simulink model "A4D_LQR"  (R2016a)
settings: Solver=VariableStepAuto  StartTime=0.0  StopTime=10.0  RelTol=1e-3
values from neighbouring files (symbols this model uses):
  A = [Y_Beta/u Y_p/u -(1-Y_r/u) g*cos(0.0872)/u ... (first row only)    [lateral.m]    (also in longitudinal.m = [X_u  X_w 0 -g; Z_u Z_w u 0; M_u+M_w_dot*Z_u M_w+M_w_dot*Z_w; rscale.m = a)
  B = [0 Y_Delta_r ... (first row only)    [lateral.m]    (also in longitudinal.m = [0; 0; M_delta+M_wdot*Z_delta; 0]; rscale.m = b)
  C = I    [lateral.m]    (also in longitudinal.m = [0 0 0 -1]; rscale.m = c)
undefined symbols (not defined in the file or in its folder): Kgain
settings Model: Creator=kumabhi  LastModifiedBy=kumabhi

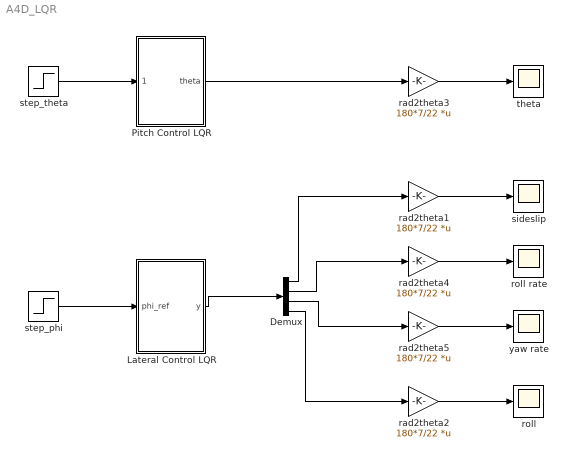
== system A4D_LQR ==
  Demux : Demux
  Lateral Control LQR : Subsystem
      mask Display: image('/home/kumabhi/Pictures/aircraft.png');
  Pitch Control LQR : Subsystem
      mask Display: image('/home/kumabhi/Pictures/aircraft.png');
  rad2theta{1..5} (5 alike) : Gain  Gain=180*7/22  Multiplication=Matrix(K*u)
  roll : Scope
  roll rate : Scope
  sideslip : Scope
  step_phi : Step  After=1.0472  SampleTime=0
  step_theta : Step  After=0.0872665  SampleTime=0
  theta : Scope
  yaw rate : Scope
  wires:
  step_theta/1 -> Pitch Control LQR/1(theta_ref)
  Pitch Control LQR/1(theta) -> rad2theta3/1
  step_phi/1 -> Lateral Control LQR/1(phi_ref)
  Lateral Control LQR/1(y) -> Demux/1
  Demux/1 -> rad2theta1/1
  rad2theta2/1 -> roll/1
  rad2theta1/1 -> sideslip/1
  rad2theta3/1 -> theta/1
  Demux/4 -> rad2theta2/1
  Demux/2 -> rad2theta4/1
  rad2theta4/1 -> roll rate/1
  Demux/3 -> rad2theta5/1
  rad2theta5/1 -> yaw rate/1

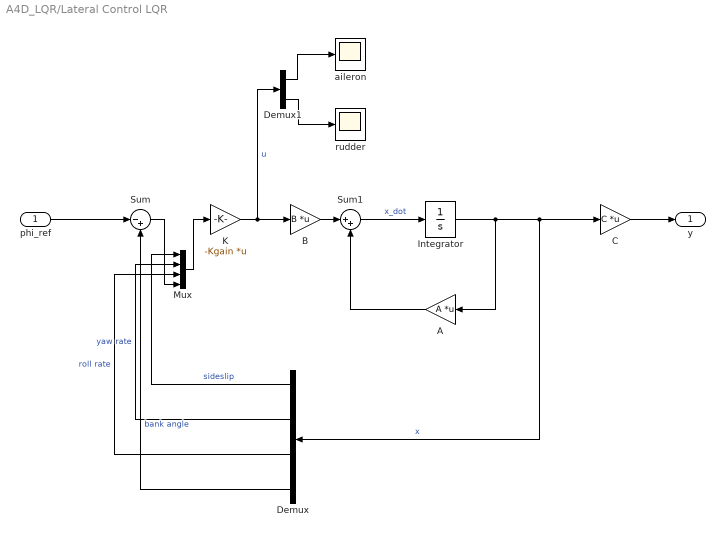
== system A4D_LQR/Lateral Control LQR ==
  phi_ref : Inport
  A : Gain  Gain=A  Multiplication=Matrix(K*u)
  B : Gain  Gain=B  Multiplication=Matrix(K*u)
  C : Gain  Gain=C  Multiplication=Matrix(K*u)
  Demux : Demux
  Demux1 : Demux  Outputs=2
  Integrator : Integrator
  K : Gain  Gain=-Kgain  Multiplication=Matrix(K*u)
  Mux : Mux
  Sum : Sum  Inputs=|-+
  Sum1 : Sum  Inputs=|++
  aileron : Scope
  rudder : Scope
  y : Outport
  wires:
  Integrator/1 -> A/1, Demux/1, C/1  "x"
  A/1 -> Sum1/2
  Sum1/1 -> Integrator/1  "x_dot"
  C/1 -> y/1
  phi_ref/1 -> Sum/1
  B/1 -> Sum1/1
  Demux/2 -> Mux/2  "yaw rate"
  Demux/3 -> Mux/3  "roll rate"
  Demux/4 -> Sum/2  "bank angle"
  Sum/1 -> Mux/4
  Mux/1 -> K/1
  K/1 -> Demux1/1, B/1  "u"
  Demux1/1 -> aileron/1
  Demux1/2 -> rudder/1
  Demux/1 -> Mux/1  "sideslip"

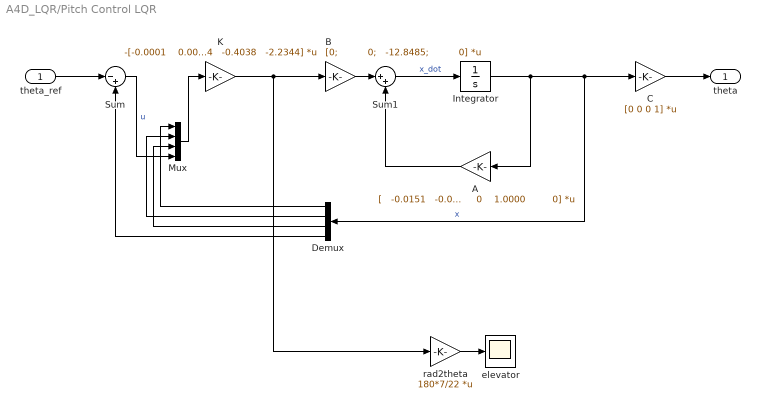
== system A4D_LQR/Pitch Control LQR ==
  theta_ref : Inport
  A : Gain  Gain=|  Multiplication=Matrix(K*u)
      | [   -0.0151   -0.0050         0   -9.8000;
      |    -0.1413   -0.8784  136.1160         0;
      |     0.0004   -0.0695   -1.4605         0;
      |          0         0    1.0000         0]
  B : Gain  Gain=|  Multiplication=Matrix(K*u)
      | [0;
      |          0;
      |   -12.8485;
      |          0]
  C : Gain  Gain=[0 0 0 1]  Multiplication=Matrix(K*u)
  Demux : Demux
  Integrator : Integrator
  K : Gain  Gain="-[-0.0001    0.0044   -0.4038   -2.2344]"  Multiplication=Matrix(K*u)
  Mux : Mux
  Sum : Sum  Inputs=|-+
  Sum1 : Sum  Inputs=|++
  elevator : Scope
  rad2theta : Gain  Gain=180*7/22  Multiplication=Matrix(K*u)
  theta : Outport
  wires:
  Integrator/1 -> A/1, Demux/1, C/1  "x"
  A/1 -> Sum1/2
  Sum1/1 -> Integrator/1  "x_dot"
  C/1 -> theta/1
  theta_ref/1 -> Sum/1
  B/1 -> Sum1/1
  Demux/1 -> Mux/1
  Demux/2 -> Mux/2
  Demux/3 -> Mux/3
  Demux/4 -> Sum/2
  Sum/1 -> Mux/4  "u"
  Mux/1 -> K/1
  K/1 -> rad2theta/1, B/1
  rad2theta/1 -> elevator/1
